simulink model "TCMSSystem"  (R2019b)
settings: configuration reference "ConfigSet_TCMSSystem_Reference" (kept outside this file)
model workspace (MAT data in the model file):
  Prm_TCMSSystem : Simulink.Parameter (value not decoded)
  SampleTime = 0.05
symbols that are objects in the model workspace (value not decoded): Prm_TCMSSystem
undefined symbols (not defined in the file): ADDIntervention, AK1Status, AK2Status, AKContactorStatus, AllDoorsClosed, AllLeftDoorsClosed, AllRightDoorsClosed, APS1Fault, APS1Isolated, APS1OutputVoltage, APS1Status, APS2Fault, APS2Isolated, APS2OutputVoltage, APS2Status, APSKAKContactor, ASCOEnd1, ASCOEnd2, ATBMode, ATCBypassMode, ATCStatusNotOK, ATOMode, ATPLowSpeedCutoutStatus, ATPMode, AuxCompressor, BatteryCurrent, BatteryIsolationContactor, BatteryTemperature, BatteryVoltage, BCG1Fault, BCG1Isolated, BCG1IsolationFailed, BCG1OutputCurrent, BCG1Status, BCG2Fault, BCG2Isolated, BCG2OutputCurrent, BCG2Status, BCGOutputVoltage, BECU1AxleLockedWheelSet1, BECU2AxleLockedWheelSet2, BECUFaulty, BECUMajorFault, BECUMinorFault, BECUStatus, BIC1Inside, BIC1Outside, BIC2Inside, BIC2Outside, Bogie, Bogie1WSPStatus, Bogie2WSPStatus, BogieFaulty, BogieIsolationStatus, BogieSupportedMass, BrakeCylinderPressureGauge, BrakeLoopCBTripped, BrakeLoopOpenTL, BrakeTrainLineStatus, BrakingDemand ... (+215)
libraries: TimersLib x257, simulink x137, LatchesLib x42, VectorOperationsLib x15, TestBenchLib x12, MathOperationsLib x2, FiltersLib x1
(part 13 of 16)

== system TCMSSystem/TCMSSystemPerVehicle/EnabledTCMSVehicle/OutputsPacking/TCMSDisplayOutputs/TCMSMessageEvents/DoorSystemFaults/Associated TCMS Fault ID121 ==
  State : Inport
  Bus Creator1 : BusCreator  Inputs=2  OutDataTypeStr=Bus: BD_TCMSSystem_Out_Vehicle_Display_Message  NonVirtualBus=on
  Constant : Constant  Value=MessageID
  Data Type Conversion : DataTypeConversion
  Message : Outport  VectorParamsAs1DForOutWhenUnconnected=off
  wires:
  Data Type Conversion/1 -> Bus Creator1/2  "MessageStatus"
  Constant/1 -> Bus Creator1/1  "MessageID"
  State/1 -> Data Type Conversion/1
  Bus Creator1/1 -> Message/1

== system TCMSSystem/TCMSSystemPerVehicle/EnabledTCMSVehicle/OutputsPacking/TCMSDisplayOutputs/TCMSMessageEvents/DoorSystemFaults/Associated TCMS Fault ID122 ==
  State : Inport
  Bus Creator1 : BusCreator  Inputs=2  OutDataTypeStr=Bus: BD_TCMSSystem_Out_Vehicle_Display_Message  NonVirtualBus=on
  Constant : Constant  Value=MessageID
  Data Type Conversion : DataTypeConversion
  Message : Outport  VectorParamsAs1DForOutWhenUnconnected=off
  wires:
  Bus Creator1/1 -> Message/1
  State/1 -> Data Type Conversion/1
  Constant/1 -> Bus Creator1/1  "MessageID"
  Data Type Conversion/1 -> Bus Creator1/2  "MessageStatus"

== system TCMSSystem/TCMSSystemPerVehicle/EnabledTCMSVehicle/OutputsPacking/TCMSDisplayOutputs/TCMSMessageEvents/DoorSystemFaults/Associated TCMS Fault ID123 ==
  State : Inport
  Bus Creator1 : BusCreator  Inputs=2  OutDataTypeStr=Bus: BD_TCMSSystem_Out_Vehicle_Display_Message  NonVirtualBus=on
  Constant : Constant  Value=MessageID
  Data Type Conversion : DataTypeConversion
  Message : Outport  VectorParamsAs1DForOutWhenUnconnected=off
  wires:
  Data Type Conversion/1 -> Bus Creator1/2  "MessageStatus"
  Constant/1 -> Bus Creator1/1  "MessageID"
  State/1 -> Data Type Conversion/1
  Bus Creator1/1 -> Message/1

== system TCMSSystem/TCMSSystemPerVehicle/EnabledTCMSVehicle/OutputsPacking/TCMSDisplayOutputs/TCMSMessageEvents/DoorSystemFaults/Associated TCMS Fault ID124 ==
  State : Inport
  Bus Creator1 : BusCreator  Inputs=2  OutDataTypeStr=Bus: BD_TCMSSystem_Out_Vehicle_Display_Message  NonVirtualBus=on
  Constant : Constant  Value=MessageID
  Data Type Conversion : DataTypeConversion
  Message : Outport  VectorParamsAs1DForOutWhenUnconnected=off
  wires:
  Data Type Conversion/1 -> Bus Creator1/2  "MessageStatus"
  Constant/1 -> Bus Creator1/1  "MessageID"
  State/1 -> Data Type Conversion/1
  Bus Creator1/1 -> Message/1

== system TCMSSystem/TCMSSystemPerVehicle/EnabledTCMSVehicle/OutputsPacking/TCMSDisplayOutputs/TCMSMessageEvents/DoorSystemFaults/Associated TCMS Fault ID125 ==
  State : Inport
  Bus Creator1 : BusCreator  Inputs=2  OutDataTypeStr=Bus: BD_TCMSSystem_Out_Vehicle_Display_Message  NonVirtualBus=on
  Constant : Constant  Value=MessageID
  Data Type Conversion : DataTypeConversion
  Message : Outport  VectorParamsAs1DForOutWhenUnconnected=off
  wires:
  Data Type Conversion/1 -> Bus Creator1/2  "MessageStatus"
  Constant/1 -> Bus Creator1/1  "MessageID"
  State/1 -> Data Type Conversion/1
  Bus Creator1/1 -> Message/1

== system TCMSSystem/TCMSSystemPerVehicle/EnabledTCMSVehicle/OutputsPacking/TCMSDisplayOutputs/TCMSMessageEvents/DoorSystemFaults/Associated TCMS Fault ID126 ==
  State : Inport
  Bus Creator1 : BusCreator  Inputs=2  OutDataTypeStr=Bus: BD_TCMSSystem_Out_Vehicle_Display_Message  NonVirtualBus=on
  Constant : Constant  Value=MessageID
  Data Type Conversion : DataTypeConversion
  Message : Outport  VectorParamsAs1DForOutWhenUnconnected=off
  wires:
  Data Type Conversion/1 -> Bus Creator1/2  "MessageStatus"
  Constant/1 -> Bus Creator1/1  "MessageID"
  State/1 -> Data Type Conversion/1
  Bus Creator1/1 -> Message/1

== system TCMSSystem/TCMSSystemPerVehicle/EnabledTCMSVehicle/OutputsPacking/TCMSDisplayOutputs/TCMSMessageEvents/DoorSystemFaults/Associated TCMS Fault ID127 ==
  State : Inport
  Bus Creator1 : BusCreator  Inputs=2  OutDataTypeStr=Bus: BD_TCMSSystem_Out_Vehicle_Display_Message  NonVirtualBus=on
  Constant : Constant  Value=MessageID
  Data Type Conversion : DataTypeConversion
  Message : Outport  VectorParamsAs1DForOutWhenUnconnected=off
  wires:
  Data Type Conversion/1 -> Bus Creator1/2  "MessageStatus"
  Constant/1 -> Bus Creator1/1  "MessageID"
  State/1 -> Data Type Conversion/1
  Bus Creator1/1 -> Message/1

== system TCMSSystem/TCMSSystemPerVehicle/EnabledTCMSVehicle/OutputsPacking/TCMSDisplayOutputs/TCMSMessageEvents/DoorSystemFaults/Associated TCMS Fault ID128 ==
  State : Inport
  Bus Creator1 : BusCreator  Inputs=2  OutDataTypeStr=Bus: BD_TCMSSystem_Out_Vehicle_Display_Message  NonVirtualBus=on
  Constant : Constant  Value=MessageID
  Data Type Conversion : DataTypeConversion
  Message : Outport  VectorParamsAs1DForOutWhenUnconnected=off
  wires:
  Bus Creator1/1 -> Message/1
  State/1 -> Data Type Conversion/1
  Constant/1 -> Bus Creator1/1  "MessageID"
  Data Type Conversion/1 -> Bus Creator1/2  "MessageStatus"

== system TCMSSystem/TCMSSystemPerVehicle/EnabledTCMSVehicle/OutputsPacking/TCMSDisplayOutputs/TCMSMessageEvents/DoorSystemFaults/Associated TCMS Fault ID129 ==
  State : Inport
  Bus Creator1 : BusCreator  Inputs=2  OutDataTypeStr=Bus: BD_TCMSSystem_Out_Vehicle_Display_Message  NonVirtualBus=on
  Constant : Constant  Value=MessageID
  Data Type Conversion : DataTypeConversion
  Message : Outport  VectorParamsAs1DForOutWhenUnconnected=off
  wires:
  Bus Creator1/1 -> Message/1
  State/1 -> Data Type Conversion/1
  Constant/1 -> Bus Creator1/1  "MessageID"
  Data Type Conversion/1 -> Bus Creator1/2  "MessageStatus"

== system TCMSSystem/TCMSSystemPerVehicle/EnabledTCMSVehicle/OutputsPacking/TCMSDisplayOutputs/TCMSMessageEvents/DoorSystemFaults/Associated TCMS Fault ID13 ==
  State : Inport
  Bus Creator1 : BusCreator  Inputs=2  OutDataTypeStr=Bus: BD_TCMSSystem_Out_Vehicle_Display_Message  NonVirtualBus=on
  Constant : Constant  Value=MessageID
  Data Type Conversion : DataTypeConversion
  Message : Outport  VectorParamsAs1DForOutWhenUnconnected=off
  wires:
  Bus Creator1/1 -> Message/1
  State/1 -> Data Type Conversion/1
  Constant/1 -> Bus Creator1/1  "MessageID"
  Data Type Conversion/1 -> Bus Creator1/2  "MessageStatus"

== system TCMSSystem/TCMSSystemPerVehicle/EnabledTCMSVehicle/OutputsPacking/TCMSDisplayOutputs/TCMSMessageEvents/DoorSystemFaults/Associated TCMS Fault ID130 ==
  State : Inport
  Bus Creator1 : BusCreator  Inputs=2  OutDataTypeStr=Bus: BD_TCMSSystem_Out_Vehicle_Display_Message  NonVirtualBus=on
  Constant : Constant  Value=MessageID
  Data Type Conversion : DataTypeConversion
  Message : Outport  VectorParamsAs1DForOutWhenUnconnected=off
  wires:
  Data Type Conversion/1 -> Bus Creator1/2  "MessageStatus"
  Constant/1 -> Bus Creator1/1  "MessageID"
  State/1 -> Data Type Conversion/1
  Bus Creator1/1 -> Message/1

== system TCMSSystem/TCMSSystemPerVehicle/EnabledTCMSVehicle/OutputsPacking/TCMSDisplayOutputs/TCMSMessageEvents/DoorSystemFaults/Associated TCMS Fault ID131 ==
  State : Inport
  Bus Creator1 : BusCreator  Inputs=2  OutDataTypeStr=Bus: BD_TCMSSystem_Out_Vehicle_Display_Message  NonVirtualBus=on
  Constant : Constant  Value=MessageID
  Data Type Conversion : DataTypeConversion
  Message : Outport  VectorParamsAs1DForOutWhenUnconnected=off
  wires:
  Data Type Conversion/1 -> Bus Creator1/2  "MessageStatus"
  Constant/1 -> Bus Creator1/1  "MessageID"
  State/1 -> Data Type Conversion/1
  Bus Creator1/1 -> Message/1

== system TCMSSystem/TCMSSystemPerVehicle/EnabledTCMSVehicle/OutputsPacking/TCMSDisplayOutputs/TCMSMessageEvents/DoorSystemFaults/Associated TCMS Fault ID132 ==
  State : Inport
  Bus Creator1 : BusCreator  Inputs=2  OutDataTypeStr=Bus: BD_TCMSSystem_Out_Vehicle_Display_Message  NonVirtualBus=on
  Constant : Constant  Value=MessageID
  Data Type Conversion : DataTypeConversion
  Message : Outport  VectorParamsAs1DForOutWhenUnconnected=off
  wires:
  Data Type Conversion/1 -> Bus Creator1/2  "MessageStatus"
  Constant/1 -> Bus Creator1/1  "MessageID"
  State/1 -> Data Type Conversion/1
  Bus Creator1/1 -> Message/1

== system TCMSSystem/TCMSSystemPerVehicle/EnabledTCMSVehicle/OutputsPacking/TCMSDisplayOutputs/TCMSMessageEvents/DoorSystemFaults/Associated TCMS Fault ID133 ==
  State : Inport
  Bus Creator1 : BusCreator  Inputs=2  OutDataTypeStr=Bus: BD_TCMSSystem_Out_Vehicle_Display_Message  NonVirtualBus=on
  Constant : Constant  Value=MessageID
  Data Type Conversion : DataTypeConversion
  Message : Outport  VectorParamsAs1DForOutWhenUnconnected=off
  wires:
  Data Type Conversion/1 -> Bus Creator1/2  "MessageStatus"
  Constant/1 -> Bus Creator1/1  "MessageID"
  State/1 -> Data Type Conversion/1
  Bus Creator1/1 -> Message/1

== system TCMSSystem/TCMSSystemPerVehicle/EnabledTCMSVehicle/OutputsPacking/TCMSDisplayOutputs/TCMSMessageEvents/DoorSystemFaults/Associated TCMS Fault ID134 ==
  State : Inport
  Bus Creator1 : BusCreator  Inputs=2  OutDataTypeStr=Bus: BD_TCMSSystem_Out_Vehicle_Display_Message  NonVirtualBus=on
  Constant : Constant  Value=MessageID
  Data Type Conversion : DataTypeConversion
  Message : Outport  VectorParamsAs1DForOutWhenUnconnected=off
  wires:
  Data Type Conversion/1 -> Bus Creator1/2  "MessageStatus"
  Constant/1 -> Bus Creator1/1  "MessageID"
  State/1 -> Data Type Conversion/1
  Bus Creator1/1 -> Message/1

== system TCMSSystem/TCMSSystemPerVehicle/EnabledTCMSVehicle/OutputsPacking/TCMSDisplayOutputs/TCMSMessageEvents/DoorSystemFaults/Associated TCMS Fault ID135 ==
  State : Inport
  Bus Creator1 : BusCreator  Inputs=2  OutDataTypeStr=Bus: BD_TCMSSystem_Out_Vehicle_Display_Message  NonVirtualBus=on
  Constant : Constant  Value=MessageID
  Data Type Conversion : DataTypeConversion
  Message : Outport  VectorParamsAs1DForOutWhenUnconnected=off
  wires:
  Bus Creator1/1 -> Message/1
  State/1 -> Data Type Conversion/1
  Constant/1 -> Bus Creator1/1  "MessageID"
  Data Type Conversion/1 -> Bus Creator1/2  "MessageStatus"

== system TCMSSystem/TCMSSystemPerVehicle/EnabledTCMSVehicle/OutputsPacking/TCMSDisplayOutputs/TCMSMessageEvents/DoorSystemFaults/Associated TCMS Fault ID14 ==
  State : Inport
  Bus Creator1 : BusCreator  Inputs=2  OutDataTypeStr=Bus: BD_TCMSSystem_Out_Vehicle_Display_Message  NonVirtualBus=on
  Constant : Constant  Value=MessageID
  Data Type Conversion : DataTypeConversion
  Message : Outport  VectorParamsAs1DForOutWhenUnconnected=off
  wires:
  Bus Creator1/1 -> Message/1
  State/1 -> Data Type Conversion/1
  Constant/1 -> Bus Creator1/1  "MessageID"
  Data Type Conversion/1 -> Bus Creator1/2  "MessageStatus"

== system TCMSSystem/TCMSSystemPerVehicle/EnabledTCMSVehicle/OutputsPacking/TCMSDisplayOutputs/TCMSMessageEvents/DoorSystemFaults/Associated TCMS Fault ID15 ==
  State : Inport
  Bus Creator1 : BusCreator  Inputs=2  OutDataTypeStr=Bus: BD_TCMSSystem_Out_Vehicle_Display_Message  NonVirtualBus=on
  Constant : Constant  Value=MessageID
  Data Type Conversion : DataTypeConversion
  Message : Outport  VectorParamsAs1DForOutWhenUnconnected=off
  wires:
  Bus Creator1/1 -> Message/1
  State/1 -> Data Type Conversion/1
  Constant/1 -> Bus Creator1/1  "MessageID"
  Data Type Conversion/1 -> Bus Creator1/2  "MessageStatus"

== system TCMSSystem/TCMSSystemPerVehicle/EnabledTCMSVehicle/OutputsPacking/TCMSDisplayOutputs/TCMSMessageEvents/DoorSystemFaults/Associated TCMS Fault ID16 ==
  State : Inport
  Bus Creator1 : BusCreator  Inputs=2  OutDataTypeStr=Bus: BD_TCMSSystem_Out_Vehicle_Display_Message  NonVirtualBus=on
  Constant : Constant  Value=MessageID
  Data Type Conversion : DataTypeConversion
  Message : Outport  VectorParamsAs1DForOutWhenUnconnected=off
  wires:
  Bus Creator1/1 -> Message/1
  State/1 -> Data Type Conversion/1
  Constant/1 -> Bus Creator1/1  "MessageID"
  Data Type Conversion/1 -> Bus Creator1/2  "MessageStatus"

== system TCMSSystem/TCMSSystemPerVehicle/EnabledTCMSVehicle/OutputsPacking/TCMSDisplayOutputs/TCMSMessageEvents/DoorSystemFaults/Associated TCMS Fault ID17 ==
  State : Inport
  Bus Creator1 : BusCreator  Inputs=2  OutDataTypeStr=Bus: BD_TCMSSystem_Out_Vehicle_Display_Message  NonVirtualBus=on
  Constant : Constant  Value=MessageID
  Data Type Conversion : DataTypeConversion
  Message : Outport  VectorParamsAs1DForOutWhenUnconnected=off
  wires:
  Bus Creator1/1 -> Message/1
  State/1 -> Data Type Conversion/1
  Constant/1 -> Bus Creator1/1  "MessageID"
  Data Type Conversion/1 -> Bus Creator1/2  "MessageStatus"

== system TCMSSystem/TCMSSystemPerVehicle/EnabledTCMSVehicle/OutputsPacking/TCMSDisplayOutputs/TCMSMessageEvents/DoorSystemFaults/Associated TCMS Fault ID18 ==
  State : Inport
  Bus Creator1 : BusCreator  Inputs=2  OutDataTypeStr=Bus: BD_TCMSSystem_Out_Vehicle_Display_Message  NonVirtualBus=on
  Constant : Constant  Value=MessageID
  Data Type Conversion : DataTypeConversion
  Message : Outport  VectorParamsAs1DForOutWhenUnconnected=off
  wires:
  Bus Creator1/1 -> Message/1
  State/1 -> Data Type Conversion/1
  Constant/1 -> Bus Creator1/1  "MessageID"
  Data Type Conversion/1 -> Bus Creator1/2  "MessageStatus"

== system TCMSSystem/TCMSSystemPerVehicle/EnabledTCMSVehicle/OutputsPacking/TCMSDisplayOutputs/TCMSMessageEvents/DoorSystemFaults/Associated TCMS Fault ID19 ==
  State : Inport
  Bus Creator1 : BusCreator  Inputs=2  OutDataTypeStr=Bus: BD_TCMSSystem_Out_Vehicle_Display_Message  NonVirtualBus=on
  Constant : Constant  Value=MessageID
  Data Type Conversion : DataTypeConversion
  Message : Outport  VectorParamsAs1DForOutWhenUnconnected=off
  wires:
  Bus Creator1/1 -> Message/1
  State/1 -> Data Type Conversion/1
  Constant/1 -> Bus Creator1/1  "MessageID"
  Data Type Conversion/1 -> Bus Creator1/2  "MessageStatus"

== system TCMSSystem/TCMSSystemPerVehicle/EnabledTCMSVehicle/OutputsPacking/TCMSDisplayOutputs/TCMSMessageEvents/DoorSystemFaults/Associated TCMS Fault ID2 ==
  State : Inport
  Bus Creator1 : BusCreator  Inputs=2  OutDataTypeStr=Bus: BD_TCMSSystem_Out_Vehicle_Display_Message  NonVirtualBus=on
  Constant : Constant  Value=MessageID
  Data Type Conversion : DataTypeConversion
  Message : Outport  VectorParamsAs1DForOutWhenUnconnected=off
  wires:
  Data Type Conversion/1 -> Bus Creator1/2  "MessageStatus"
  Constant/1 -> Bus Creator1/1  "MessageID"
  State/1 -> Data Type Conversion/1
  Bus Creator1/1 -> Message/1

== system TCMSSystem/TCMSSystemPerVehicle/EnabledTCMSVehicle/OutputsPacking/TCMSDisplayOutputs/TCMSMessageEvents/DoorSystemFaults/Associated TCMS Fault ID20 ==
  State : Inport
  Bus Creator1 : BusCreator  Inputs=2  OutDataTypeStr=Bus: BD_TCMSSystem_Out_Vehicle_Display_Message  NonVirtualBus=on
  Constant : Constant  Value=MessageID
  Data Type Conversion : DataTypeConversion
  Message : Outport  VectorParamsAs1DForOutWhenUnconnected=off
  wires:
  Data Type Conversion/1 -> Bus Creator1/2  "MessageStatus"
  Constant/1 -> Bus Creator1/1  "MessageID"
  State/1 -> Data Type Conversion/1
  Bus Creator1/1 -> Message/1

== system TCMSSystem/TCMSSystemPerVehicle/EnabledTCMSVehicle/OutputsPacking/TCMSDisplayOutputs/TCMSMessageEvents/DoorSystemFaults/Associated TCMS Fault ID21 ==
  State : Inport
  Bus Creator1 : BusCreator  Inputs=2  OutDataTypeStr=Bus: BD_TCMSSystem_Out_Vehicle_Display_Message  NonVirtualBus=on
  Constant : Constant  Value=MessageID
  Data Type Conversion : DataTypeConversion
  Message : Outport  VectorParamsAs1DForOutWhenUnconnected=off
  wires:
  Data Type Conversion/1 -> Bus Creator1/2  "MessageStatus"
  Constant/1 -> Bus Creator1/1  "MessageID"
  State/1 -> Data Type Conversion/1
  Bus Creator1/1 -> Message/1

== system TCMSSystem/TCMSSystemPerVehicle/EnabledTCMSVehicle/OutputsPacking/TCMSDisplayOutputs/TCMSMessageEvents/DoorSystemFaults/Associated TCMS Fault ID22 ==
  State : Inport
  Bus Creator1 : BusCreator  Inputs=2  OutDataTypeStr=Bus: BD_TCMSSystem_Out_Vehicle_Display_Message  NonVirtualBus=on
  Constant : Constant  Value=MessageID
  Data Type Conversion : DataTypeConversion
  Message : Outport  VectorParamsAs1DForOutWhenUnconnected=off
  wires:
  Data Type Conversion/1 -> Bus Creator1/2  "MessageStatus"
  Constant/1 -> Bus Creator1/1  "MessageID"
  State/1 -> Data Type Conversion/1
  Bus Creator1/1 -> Message/1

== system TCMSSystem/TCMSSystemPerVehicle/EnabledTCMSVehicle/OutputsPacking/TCMSDisplayOutputs/TCMSMessageEvents/DoorSystemFaults/Associated TCMS Fault ID23 ==
  State : Inport
  Bus Creator1 : BusCreator  Inputs=2  OutDataTypeStr=Bus: BD_TCMSSystem_Out_Vehicle_Display_Message  NonVirtualBus=on
  Constant : Constant  Value=MessageID
  Data Type Conversion : DataTypeConversion
  Message : Outport  VectorParamsAs1DForOutWhenUnconnected=off
  wires:
  Data Type Conversion/1 -> Bus Creator1/2  "MessageStatus"
  Constant/1 -> Bus Creator1/1  "MessageID"
  State/1 -> Data Type Conversion/1
  Bus Creator1/1 -> Message/1

== system TCMSSystem/TCMSSystemPerVehicle/EnabledTCMSVehicle/OutputsPacking/TCMSDisplayOutputs/TCMSMessageEvents/DoorSystemFaults/Associated TCMS Fault ID24 ==
  State : Inport
  Bus Creator1 : BusCreator  Inputs=2  OutDataTypeStr=Bus: BD_TCMSSystem_Out_Vehicle_Display_Message  NonVirtualBus=on
  Constant : Constant  Value=MessageID
  Data Type Conversion : DataTypeConversion
  Message : Outport  VectorParamsAs1DForOutWhenUnconnected=off
  wires:
  Data Type Conversion/1 -> Bus Creator1/2  "MessageStatus"
  Constant/1 -> Bus Creator1/1  "MessageID"
  State/1 -> Data Type Conversion/1
  Bus Creator1/1 -> Message/1

== system TCMSSystem/TCMSSystemPerVehicle/EnabledTCMSVehicle/OutputsPacking/TCMSDisplayOutputs/TCMSMessageEvents/DoorSystemFaults/Associated TCMS Fault ID25 ==
  State : Inport
  Bus Creator1 : BusCreator  Inputs=2  OutDataTypeStr=Bus: BD_TCMSSystem_Out_Vehicle_Display_Message  NonVirtualBus=on
  Constant : Constant  Value=MessageID
  Data Type Conversion : DataTypeConversion
  Message : Outport  VectorParamsAs1DForOutWhenUnconnected=off
  wires:
  Data Type Conversion/1 -> Bus Creator1/2  "MessageStatus"
  Constant/1 -> Bus Creator1/1  "MessageID"
  State/1 -> Data Type Conversion/1
  Bus Creator1/1 -> Message/1

== system TCMSSystem/TCMSSystemPerVehicle/EnabledTCMSVehicle/OutputsPacking/TCMSDisplayOutputs/TCMSMessageEvents/DoorSystemFaults/Associated TCMS Fault ID26 ==
  State : Inport
  Bus Creator1 : BusCreator  Inputs=2  OutDataTypeStr=Bus: BD_TCMSSystem_Out_Vehicle_Display_Message  NonVirtualBus=on
  Constant : Constant  Value=MessageID
  Data Type Conversion : DataTypeConversion
  Message : Outport  VectorParamsAs1DForOutWhenUnconnected=off
  wires:
  Data Type Conversion/1 -> Bus Creator1/2  "MessageStatus"
  Constant/1 -> Bus Creator1/1  "MessageID"
  State/1 -> Data Type Conversion/1
  Bus Creator1/1 -> Message/1

== system TCMSSystem/TCMSSystemPerVehicle/EnabledTCMSVehicle/OutputsPacking/TCMSDisplayOutputs/TCMSMessageEvents/DoorSystemFaults/Associated TCMS Fault ID27 ==
  State : Inport
  Bus Creator1 : BusCreator  Inputs=2  OutDataTypeStr=Bus: BD_TCMSSystem_Out_Vehicle_Display_Message  NonVirtualBus=on
  Constant : Constant  Value=MessageID
  Data Type Conversion : DataTypeConversion
  Message : Outport  VectorParamsAs1DForOutWhenUnconnected=off
  wires:
  Data Type Conversion/1 -> Bus Creator1/2  "MessageStatus"
  Constant/1 -> Bus Creator1/1  "MessageID"
  State/1 -> Data Type Conversion/1
  Bus Creator1/1 -> Message/1

== system TCMSSystem/TCMSSystemPerVehicle/EnabledTCMSVehicle/OutputsPacking/TCMSDisplayOutputs/TCMSMessageEvents/DoorSystemFaults/Associated TCMS Fault ID28 ==
  State : Inport
  Bus Creator1 : BusCreator  Inputs=2  OutDataTypeStr=Bus: BD_TCMSSystem_Out_Vehicle_Display_Message  NonVirtualBus=on
  Constant : Constant  Value=MessageID
  Data Type Conversion : DataTypeConversion
  Message : Outport  VectorParamsAs1DForOutWhenUnconnected=off
  wires:
  Data Type Conversion/1 -> Bus Creator1/2  "MessageStatus"
  Constant/1 -> Bus Creator1/1  "MessageID"
  State/1 -> Data Type Conversion/1
  Bus Creator1/1 -> Message/1

== system TCMSSystem/TCMSSystemPerVehicle/EnabledTCMSVehicle/OutputsPacking/TCMSDisplayOutputs/TCMSMessageEvents/DoorSystemFaults/Associated TCMS Fault ID29 ==
  State : Inport
  Bus Creator1 : BusCreator  Inputs=2  OutDataTypeStr=Bus: BD_TCMSSystem_Out_Vehicle_Display_Message  NonVirtualBus=on
  Constant : Constant  Value=MessageID
  Data Type Conversion : DataTypeConversion
  Message : Outport  VectorParamsAs1DForOutWhenUnconnected=off
  wires:
  Data Type Conversion/1 -> Bus Creator1/2  "MessageStatus"
  Constant/1 -> Bus Creator1/1  "MessageID"
  State/1 -> Data Type Conversion/1
  Bus Creator1/1 -> Message/1

== system TCMSSystem/TCMSSystemPerVehicle/EnabledTCMSVehicle/OutputsPacking/TCMSDisplayOutputs/TCMSMessageEvents/DoorSystemFaults/Associated TCMS Fault ID3 ==
  State : Inport
  Bus Creator1 : BusCreator  Inputs=2  OutDataTypeStr=Bus: BD_TCMSSystem_Out_Vehicle_Display_Message  NonVirtualBus=on
  Constant : Constant  Value=MessageID
  Data Type Conversion : DataTypeConversion
  Message : Outport  VectorParamsAs1DForOutWhenUnconnected=off
  wires:
  Data Type Conversion/1 -> Bus Creator1/2  "MessageStatus"
  Constant/1 -> Bus Creator1/1  "MessageID"
  State/1 -> Data Type Conversion/1
  Bus Creator1/1 -> Message/1

== system TCMSSystem/TCMSSystemPerVehicle/EnabledTCMSVehicle/OutputsPacking/TCMSDisplayOutputs/TCMSMessageEvents/DoorSystemFaults/Associated TCMS Fault ID30 ==
  State : Inport
  Bus Creator1 : BusCreator  Inputs=2  OutDataTypeStr=Bus: BD_TCMSSystem_Out_Vehicle_Display_Message  NonVirtualBus=on
  Constant : Constant  Value=MessageID
  Data Type Conversion : DataTypeConversion
  Message : Outport  VectorParamsAs1DForOutWhenUnconnected=off
  wires:
  Bus Creator1/1 -> Message/1
  State/1 -> Data Type Conversion/1
  Constant/1 -> Bus Creator1/1  "MessageID"
  Data Type Conversion/1 -> Bus Creator1/2  "MessageStatus"

== system TCMSSystem/TCMSSystemPerVehicle/EnabledTCMSVehicle/OutputsPacking/TCMSDisplayOutputs/TCMSMessageEvents/DoorSystemFaults/Associated TCMS Fault ID31 ==
  State : Inport
  Bus Creator1 : BusCreator  Inputs=2  OutDataTypeStr=Bus: BD_TCMSSystem_Out_Vehicle_Display_Message  NonVirtualBus=on
  Constant : Constant  Value=MessageID
  Data Type Conversion : DataTypeConversion
  Message : Outport  VectorParamsAs1DForOutWhenUnconnected=off
  wires:
  Bus Creator1/1 -> Message/1
  State/1 -> Data Type Conversion/1
  Constant/1 -> Bus Creator1/1  "MessageID"
  Data Type Conversion/1 -> Bus Creator1/2  "MessageStatus"

== system TCMSSystem/TCMSSystemPerVehicle/EnabledTCMSVehicle/OutputsPacking/TCMSDisplayOutputs/TCMSMessageEvents/DoorSystemFaults/Associated TCMS Fault ID32 ==
  State : Inport
  Bus Creator1 : BusCreator  Inputs=2  OutDataTypeStr=Bus: BD_TCMSSystem_Out_Vehicle_Display_Message  NonVirtualBus=on
  Constant : Constant  Value=MessageID
  Data Type Conversion : DataTypeConversion
  Message : Outport  VectorParamsAs1DForOutWhenUnconnected=off
  wires:
  Bus Creator1/1 -> Message/1
  State/1 -> Data Type Conversion/1
  Constant/1 -> Bus Creator1/1  "MessageID"
  Data Type Conversion/1 -> Bus Creator1/2  "MessageStatus"

== system TCMSSystem/TCMSSystemPerVehicle/EnabledTCMSVehicle/OutputsPacking/TCMSDisplayOutputs/TCMSMessageEvents/DoorSystemFaults/Associated TCMS Fault ID33 ==
  State : Inport
  Bus Creator1 : BusCreator  Inputs=2  OutDataTypeStr=Bus: BD_TCMSSystem_Out_Vehicle_Display_Message  NonVirtualBus=on
  Constant : Constant  Value=MessageID
  Data Type Conversion : DataTypeConversion
  Message : Outport  VectorParamsAs1DForOutWhenUnconnected=off
  wires:
  Bus Creator1/1 -> Message/1
  State/1 -> Data Type Conversion/1
  Constant/1 -> Bus Creator1/1  "MessageID"
  Data Type Conversion/1 -> Bus Creator1/2  "MessageStatus"

== system TCMSSystem/TCMSSystemPerVehicle/EnabledTCMSVehicle/OutputsPacking/TCMSDisplayOutputs/TCMSMessageEvents/DoorSystemFaults/Associated TCMS Fault ID34 ==
  State : Inport
  Bus Creator1 : BusCreator  Inputs=2  OutDataTypeStr=Bus: BD_TCMSSystem_Out_Vehicle_Display_Message  NonVirtualBus=on
  Constant : Constant  Value=MessageID
  Data Type Conversion : DataTypeConversion
  Message : Outport  VectorParamsAs1DForOutWhenUnconnected=off
  wires:
  Bus Creator1/1 -> Message/1
  State/1 -> Data Type Conversion/1
  Constant/1 -> Bus Creator1/1  "MessageID"
  Data Type Conversion/1 -> Bus Creator1/2  "MessageStatus"

== system TCMSSystem/TCMSSystemPerVehicle/EnabledTCMSVehicle/OutputsPacking/TCMSDisplayOutputs/TCMSMessageEvents/DoorSystemFaults/Associated TCMS Fault ID35 ==
  State : Inport
  Bus Creator1 : BusCreator  Inputs=2  OutDataTypeStr=Bus: BD_TCMSSystem_Out_Vehicle_Display_Message  NonVirtualBus=on
  Constant : Constant  Value=MessageID
  Data Type Conversion : DataTypeConversion
  Message : Outport  VectorParamsAs1DForOutWhenUnconnected=off
  wires:
  Bus Creator1/1 -> Message/1
  State/1 -> Data Type Conversion/1
  Constant/1 -> Bus Creator1/1  "MessageID"
  Data Type Conversion/1 -> Bus Creator1/2  "MessageStatus"

== system TCMSSystem/TCMSSystemPerVehicle/EnabledTCMSVehicle/OutputsPacking/TCMSDisplayOutputs/TCMSMessageEvents/DoorSystemFaults/Associated TCMS Fault ID36 ==
  State : Inport
  Bus Creator1 : BusCreator  Inputs=2  OutDataTypeStr=Bus: BD_TCMSSystem_Out_Vehicle_Display_Message  NonVirtualBus=on
  Constant : Constant  Value=MessageID
  Data Type Conversion : DataTypeConversion
  Message : Outport  VectorParamsAs1DForOutWhenUnconnected=off
  wires:
  Bus Creator1/1 -> Message/1
  State/1 -> Data Type Conversion/1
  Constant/1 -> Bus Creator1/1  "MessageID"
  Data Type Conversion/1 -> Bus Creator1/2  "MessageStatus"

== system TCMSSystem/TCMSSystemPerVehicle/EnabledTCMSVehicle/OutputsPacking/TCMSDisplayOutputs/TCMSMessageEvents/DoorSystemFaults/Associated TCMS Fault ID37 ==
  State : Inport
  Bus Creator1 : BusCreator  Inputs=2  OutDataTypeStr=Bus: BD_TCMSSystem_Out_Vehicle_Display_Message  NonVirtualBus=on
  Constant : Constant  Value=MessageID
  Data Type Conversion : DataTypeConversion
  Message : Outport  VectorParamsAs1DForOutWhenUnconnected=off
  wires:
  Bus Creator1/1 -> Message/1
  State/1 -> Data Type Conversion/1
  Constant/1 -> Bus Creator1/1  "MessageID"
  Data Type Conversion/1 -> Bus Creator1/2  "MessageStatus"

== system TCMSSystem/TCMSSystemPerVehicle/EnabledTCMSVehicle/OutputsPacking/TCMSDisplayOutputs/TCMSMessageEvents/DoorSystemFaults/Associated TCMS Fault ID38 ==
  State : Inport
  Bus Creator1 : BusCreator  Inputs=2  OutDataTypeStr=Bus: BD_TCMSSystem_Out_Vehicle_Display_Message  NonVirtualBus=on
  Constant : Constant  Value=MessageID
  Data Type Conversion : DataTypeConversion
  Message : Outport  VectorParamsAs1DForOutWhenUnconnected=off
  wires:
  Bus Creator1/1 -> Message/1
  State/1 -> Data Type Conversion/1
  Constant/1 -> Bus Creator1/1  "MessageID"
  Data Type Conversion/1 -> Bus Creator1/2  "MessageStatus"

== system TCMSSystem/TCMSSystemPerVehicle/EnabledTCMSVehicle/OutputsPacking/TCMSDisplayOutputs/TCMSMessageEvents/DoorSystemFaults/Associated TCMS Fault ID4 ==
  State : Inport
  Bus Creator1 : BusCreator  Inputs=2  OutDataTypeStr=Bus: BD_TCMSSystem_Out_Vehicle_Display_Message  NonVirtualBus=on
  Constant : Constant  Value=MessageID
  Data Type Conversion : DataTypeConversion
  Message : Outport  VectorParamsAs1DForOutWhenUnconnected=off
  wires:
  Data Type Conversion/1 -> Bus Creator1/2  "MessageStatus"
  Constant/1 -> Bus Creator1/1  "MessageID"
  State/1 -> Data Type Conversion/1
  Bus Creator1/1 -> Message/1

== system TCMSSystem/TCMSSystemPerVehicle/EnabledTCMSVehicle/OutputsPacking/TCMSDisplayOutputs/TCMSMessageEvents/DoorSystemFaults/Associated TCMS Fault ID5 ==
  State : Inport
  Bus Creator1 : BusCreator  Inputs=2  OutDataTypeStr=Bus: BD_TCMSSystem_Out_Vehicle_Display_Message  NonVirtualBus=on
  Constant : Constant  Value=MessageID
  Data Type Conversion : DataTypeConversion
  Message : Outport  VectorParamsAs1DForOutWhenUnconnected=off
  wires:
  Data Type Conversion/1 -> Bus Creator1/2  "MessageStatus"
  Constant/1 -> Bus Creator1/1  "MessageID"
  State/1 -> Data Type Conversion/1
  Bus Creator1/1 -> Message/1

== system TCMSSystem/TCMSSystemPerVehicle/EnabledTCMSVehicle/OutputsPacking/TCMSDisplayOutputs/TCMSMessageEvents/DoorSystemFaults/Associated TCMS Fault ID6 ==
  State : Inport
  Bus Creator1 : BusCreator  Inputs=2  OutDataTypeStr=Bus: BD_TCMSSystem_Out_Vehicle_Display_Message  NonVirtualBus=on
  Constant : Constant  Value=MessageID
  Data Type Conversion : DataTypeConversion
  Message : Outport  VectorParamsAs1DForOutWhenUnconnected=off
  wires:
  Data Type Conversion/1 -> Bus Creator1/2  "MessageStatus"
  Constant/1 -> Bus Creator1/1  "MessageID"
  State/1 -> Data Type Conversion/1
  Bus Creator1/1 -> Message/1

== system TCMSSystem/TCMSSystemPerVehicle/EnabledTCMSVehicle/OutputsPacking/TCMSDisplayOutputs/TCMSMessageEvents/DoorSystemFaults/Associated TCMS Fault ID7 ==
  State : Inport
  Bus Creator1 : BusCreator  Inputs=2  OutDataTypeStr=Bus: BD_TCMSSystem_Out_Vehicle_Display_Message  NonVirtualBus=on
  Constant : Constant  Value=MessageID
  Data Type Conversion : DataTypeConversion
  Message : Outport  VectorParamsAs1DForOutWhenUnconnected=off
  wires:
  Data Type Conversion/1 -> Bus Creator1/2  "MessageStatus"
  Constant/1 -> Bus Creator1/1  "MessageID"
  State/1 -> Data Type Conversion/1
  Bus Creator1/1 -> Message/1

== system TCMSSystem/TCMSSystemPerVehicle/EnabledTCMSVehicle/OutputsPacking/TCMSDisplayOutputs/TCMSMessageEvents/DoorSystemFaults/Associated TCMS Fault ID8 ==
  State : Inport
  Bus Creator1 : BusCreator  Inputs=2  OutDataTypeStr=Bus: BD_TCMSSystem_Out_Vehicle_Display_Message  NonVirtualBus=on
  Constant : Constant  Value=MessageID
  Data Type Conversion : DataTypeConversion
  Message : Outport  VectorParamsAs1DForOutWhenUnconnected=off
  wires:
  Data Type Conversion/1 -> Bus Creator1/2  "MessageStatus"
  Constant/1 -> Bus Creator1/1  "MessageID"
  State/1 -> Data Type Conversion/1
  Bus Creator1/1 -> Message/1

== system TCMSSystem/TCMSSystemPerVehicle/EnabledTCMSVehicle/OutputsPacking/TCMSDisplayOutputs/TCMSMessageEvents/DoorSystemFaults/Associated TCMS Fault ID9 ==
  State : Inport
  Bus Creator1 : BusCreator  Inputs=2  OutDataTypeStr=Bus: BD_TCMSSystem_Out_Vehicle_Display_Message  NonVirtualBus=on
  Constant : Constant  Value=MessageID
  Data Type Conversion : DataTypeConversion
  Message : Outport  VectorParamsAs1DForOutWhenUnconnected=off
  wires:
  Data Type Conversion/1 -> Bus Creator1/2  "MessageStatus"
  Constant/1 -> Bus Creator1/1  "MessageID"
  State/1 -> Data Type Conversion/1
  Bus Creator1/1 -> Message/1

== system TCMSSystem/TCMSSystemPerVehicle/EnabledTCMSVehicle/OutputsPacking/TCMSDisplayOutputs/TCMSMessageEvents/ElectricalSystemFaults/Associated TCMS Fault ID1 ==
  State : Inport
  Bus Creator1 : BusCreator  Inputs=2  OutDataTypeStr=Bus: BD_TCMSSystem_Out_Vehicle_Display_Message  NonVirtualBus=on
  Constant : Constant  Value=MessageID
  Data Type Conversion : DataTypeConversion
  Message : Outport  VectorParamsAs1DForOutWhenUnconnected=off
  wires:
  Data Type Conversion/1 -> Bus Creator1/2  "MessageStatus"
  Constant/1 -> Bus Creator1/1  "MessageID"
  State/1 -> Data Type Conversion/1
  Bus Creator1/1 -> Message/1

== system TCMSSystem/TCMSSystemPerVehicle/EnabledTCMSVehicle/OutputsPacking/TCMSDisplayOutputs/TCMSMessageEvents/ElectricalSystemFaults/Associated TCMS Fault ID10 ==
  State : Inport
  Bus Creator1 : BusCreator  Inputs=2  OutDataTypeStr=Bus: BD_TCMSSystem_Out_Vehicle_Display_Message  NonVirtualBus=on
  Constant : Constant  Value=MessageID
  Data Type Conversion : DataTypeConversion
  Message : Outport  VectorParamsAs1DForOutWhenUnconnected=off
  wires:
  Data Type Conversion/1 -> Bus Creator1/2  "MessageStatus"
  Constant/1 -> Bus Creator1/1  "MessageID"
  State/1 -> Data Type Conversion/1
  Bus Creator1/1 -> Message/1

== system TCMSSystem/TCMSSystemPerVehicle/EnabledTCMSVehicle/OutputsPacking/TCMSDisplayOutputs/TCMSMessageEvents/ElectricalSystemFaults/Associated TCMS Fault ID11 ==
  State : Inport
  Bus Creator1 : BusCreator  Inputs=2  OutDataTypeStr=Bus: BD_TCMSSystem_Out_Vehicle_Display_Message  NonVirtualBus=on
  Constant : Constant  Value=MessageID
  Data Type Conversion : DataTypeConversion
  Message : Outport  VectorParamsAs1DForOutWhenUnconnected=off
  wires:
  Bus Creator1/1 -> Message/1
  State/1 -> Data Type Conversion/1
  Constant/1 -> Bus Creator1/1  "MessageID"
  Data Type Conversion/1 -> Bus Creator1/2  "MessageStatus"

== system TCMSSystem/TCMSSystemPerVehicle/EnabledTCMSVehicle/OutputsPacking/TCMSDisplayOutputs/TCMSMessageEvents/ElectricalSystemFaults/Associated TCMS Fault ID12 ==
  State : Inport
  Bus Creator1 : BusCreator  Inputs=2  OutDataTypeStr=Bus: BD_TCMSSystem_Out_Vehicle_Display_Message  NonVirtualBus=on
  Constant : Constant  Value=MessageID
  Data Type Conversion : DataTypeConversion
  Message : Outport  VectorParamsAs1DForOutWhenUnconnected=off
  wires:
  Bus Creator1/1 -> Message/1
  State/1 -> Data Type Conversion/1
  Constant/1 -> Bus Creator1/1  "MessageID"
  Data Type Conversion/1 -> Bus Creator1/2  "MessageStatus"

== system TCMSSystem/TCMSSystemPerVehicle/EnabledTCMSVehicle/OutputsPacking/TCMSDisplayOutputs/TCMSMessageEvents/ElectricalSystemFaults/Associated TCMS Fault ID13 ==
  State : Inport
  Bus Creator1 : BusCreator  Inputs=2  OutDataTypeStr=Bus: BD_TCMSSystem_Out_Vehicle_Display_Message  NonVirtualBus=on
  Constant : Constant  Value=MessageID
  Data Type Conversion : DataTypeConversion
  Message : Outport  VectorParamsAs1DForOutWhenUnconnected=off
  wires:
  Data Type Conversion/1 -> Bus Creator1/2  "MessageStatus"
  Constant/1 -> Bus Creator1/1  "MessageID"
  State/1 -> Data Type Conversion/1
  Bus Creator1/1 -> Message/1

== system TCMSSystem/TCMSSystemPerVehicle/EnabledTCMSVehicle/OutputsPacking/TCMSDisplayOutputs/TCMSMessageEvents/ElectricalSystemFaults/Associated TCMS Fault ID14 ==
  State : Inport
  Bus Creator1 : BusCreator  Inputs=2  OutDataTypeStr=Bus: BD_TCMSSystem_Out_Vehicle_Display_Message  NonVirtualBus=on
  Constant : Constant  Value=MessageID
  Data Type Conversion : DataTypeConversion
  Message : Outport  VectorParamsAs1DForOutWhenUnconnected=off
  wires:
  Bus Creator1/1 -> Message/1
  State/1 -> Data Type Conversion/1
  Constant/1 -> Bus Creator1/1  "MessageID"
  Data Type Conversion/1 -> Bus Creator1/2  "MessageStatus"

== system TCMSSystem/TCMSSystemPerVehicle/EnabledTCMSVehicle/OutputsPacking/TCMSDisplayOutputs/TCMSMessageEvents/ElectricalSystemFaults/Associated TCMS Fault ID15 ==
  State : Inport
  Bus Creator1 : BusCreator  Inputs=2  OutDataTypeStr=Bus: BD_TCMSSystem_Out_Vehicle_Display_Message  NonVirtualBus=on
  Constant : Constant  Value=MessageID
  Data Type Conversion : DataTypeConversion
  Message : Outport  VectorParamsAs1DForOutWhenUnconnected=off
  wires:
  Data Type Conversion/1 -> Bus Creator1/2  "MessageStatus"
  Constant/1 -> Bus Creator1/1  "MessageID"
  State/1 -> Data Type Conversion/1
  Bus Creator1/1 -> Message/1

== system TCMSSystem/TCMSSystemPerVehicle/EnabledTCMSVehicle/OutputsPacking/TCMSDisplayOutputs/TCMSMessageEvents/ElectricalSystemFaults/Associated TCMS Fault ID16 ==
  State : Inport
  Bus Creator1 : BusCreator  Inputs=2  OutDataTypeStr=Bus: BD_TCMSSystem_Out_Vehicle_Display_Message  NonVirtualBus=on
  Constant : Constant  Value=MessageID
  Data Type Conversion : DataTypeConversion
  Message : Outport  VectorParamsAs1DForOutWhenUnconnected=off
  wires:
  Bus Creator1/1 -> Message/1
  State/1 -> Data Type Conversion/1
  Constant/1 -> Bus Creator1/1  "MessageID"
  Data Type Conversion/1 -> Bus Creator1/2  "MessageStatus"

== system TCMSSystem/TCMSSystemPerVehicle/EnabledTCMSVehicle/OutputsPacking/TCMSDisplayOutputs/TCMSMessageEvents/ElectricalSystemFaults/Associated TCMS Fault ID17 ==
  State : Inport
  Bus Creator1 : BusCreator  Inputs=2  OutDataTypeStr=Bus: BD_TCMSSystem_Out_Vehicle_Display_Message  NonVirtualBus=on
  Constant : Constant  Value=MessageID
  Data Type Conversion : DataTypeConversion
  Message : Outport  VectorParamsAs1DForOutWhenUnconnected=off
  wires:
  Data Type Conversion/1 -> Bus Creator1/2  "MessageStatus"
  Constant/1 -> Bus Creator1/1  "MessageID"
  State/1 -> Data Type Conversion/1
  Bus Creator1/1 -> Message/1

== system TCMSSystem/TCMSSystemPerVehicle/EnabledTCMSVehicle/OutputsPacking/TCMSDisplayOutputs/TCMSMessageEvents/ElectricalSystemFaults/Associated TCMS Fault ID18 ==
  State : Inport
  Bus Creator1 : BusCreator  Inputs=2  OutDataTypeStr=Bus: BD_TCMSSystem_Out_Vehicle_Display_Message  NonVirtualBus=on
  Constant : Constant  Value=MessageID
  Data Type Conversion : DataTypeConversion
  Message : Outport  VectorParamsAs1DForOutWhenUnconnected=off
  wires:
  Data Type Conversion/1 -> Bus Creator1/2  "MessageStatus"
  Constant/1 -> Bus Creator1/1  "MessageID"
  State/1 -> Data Type Conversion/1
  Bus Creator1/1 -> Message/1

== system TCMSSystem/TCMSSystemPerVehicle/EnabledTCMSVehicle/OutputsPacking/TCMSDisplayOutputs/TCMSMessageEvents/ElectricalSystemFaults/Associated TCMS Fault ID19 ==
  State : Inport
  Bus Creator1 : BusCreator  Inputs=2  OutDataTypeStr=Bus: BD_TCMSSystem_Out_Vehicle_Display_Message  NonVirtualBus=on
  Constant : Constant  Value=MessageID
  Data Type Conversion : DataTypeConversion
  Message : Outport  VectorParamsAs1DForOutWhenUnconnected=off
  wires:
  Bus Creator1/1 -> Message/1
  State/1 -> Data Type Conversion/1
  Constant/1 -> Bus Creator1/1  "MessageID"
  Data Type Conversion/1 -> Bus Creator1/2  "MessageStatus"

== system TCMSSystem/TCMSSystemPerVehicle/EnabledTCMSVehicle/OutputsPacking/TCMSDisplayOutputs/TCMSMessageEvents/ElectricalSystemFaults/Associated TCMS Fault ID2 ==
  State : Inport
  Bus Creator1 : BusCreator  Inputs=2  OutDataTypeStr=Bus: BD_TCMSSystem_Out_Vehicle_Display_Message  NonVirtualBus=on
  Constant : Constant  Value=MessageID
  Data Type Conversion : DataTypeConversion
  Message : Outport  VectorParamsAs1DForOutWhenUnconnected=off
  wires:
  Bus Creator1/1 -> Message/1
  State/1 -> Data Type Conversion/1
  Constant/1 -> Bus Creator1/1  "MessageID"
  Data Type Conversion/1 -> Bus Creator1/2  "MessageStatus"

== system TCMSSystem/TCMSSystemPerVehicle/EnabledTCMSVehicle/OutputsPacking/TCMSDisplayOutputs/TCMSMessageEvents/ElectricalSystemFaults/Associated TCMS Fault ID20 ==
  State : Inport
  Bus Creator1 : BusCreator  Inputs=2  OutDataTypeStr=Bus: BD_TCMSSystem_Out_Vehicle_Display_Message  NonVirtualBus=on
  Constant : Constant  Value=MessageID
  Data Type Conversion : DataTypeConversion
  Message : Outport  VectorParamsAs1DForOutWhenUnconnected=off
  wires:
  Data Type Conversion/1 -> Bus Creator1/2  "MessageStatus"
  Constant/1 -> Bus Creator1/1  "MessageID"
  State/1 -> Data Type Conversion/1
  Bus Creator1/1 -> Message/1

== system TCMSSystem/TCMSSystemPerVehicle/EnabledTCMSVehicle/OutputsPacking/TCMSDisplayOutputs/TCMSMessageEvents/ElectricalSystemFaults/Associated TCMS Fault ID21 ==
  State : Inport
  Bus Creator1 : BusCreator  Inputs=2  OutDataTypeStr=Bus: BD_TCMSSystem_Out_Vehicle_Display_Message  NonVirtualBus=on
  Constant : Constant  Value=MessageID
  Data Type Conversion : DataTypeConversion
  Message : Outport  VectorParamsAs1DForOutWhenUnconnected=off
  wires:
  Bus Creator1/1 -> Message/1
  State/1 -> Data Type Conversion/1
  Constant/1 -> Bus Creator1/1  "MessageID"
  Data Type Conversion/1 -> Bus Creator1/2  "MessageStatus"

== system TCMSSystem/TCMSSystemPerVehicle/EnabledTCMSVehicle/OutputsPacking/TCMSDisplayOutputs/TCMSMessageEvents/ElectricalSystemFaults/Associated TCMS Fault ID22 ==
  State : Inport
  Bus Creator1 : BusCreator  Inputs=2  OutDataTypeStr=Bus: BD_TCMSSystem_Out_Vehicle_Display_Message  NonVirtualBus=on
  Constant : Constant  Value=MessageID
  Data Type Conversion : DataTypeConversion
  Message : Outport  VectorParamsAs1DForOutWhenUnconnected=off
  wires:
  Bus Creator1/1 -> Message/1
  State/1 -> Data Type Conversion/1
  Constant/1 -> Bus Creator1/1  "MessageID"
  Data Type Conversion/1 -> Bus Creator1/2  "MessageStatus"

== system TCMSSystem/TCMSSystemPerVehicle/EnabledTCMSVehicle/OutputsPacking/TCMSDisplayOutputs/TCMSMessageEvents/ElectricalSystemFaults/Associated TCMS Fault ID23 ==
  State : Inport
  Bus Creator1 : BusCreator  Inputs=2  OutDataTypeStr=Bus: BD_TCMSSystem_Out_Vehicle_Display_Message  NonVirtualBus=on
  Constant : Constant  Value=MessageID
  Data Type Conversion : DataTypeConversion
  Message : Outport  VectorParamsAs1DForOutWhenUnconnected=off
  wires:
  Bus Creator1/1 -> Message/1
  State/1 -> Data Type Conversion/1
  Constant/1 -> Bus Creator1/1  "MessageID"
  Data Type Conversion/1 -> Bus Creator1/2  "MessageStatus"

== system TCMSSystem/TCMSSystemPerVehicle/EnabledTCMSVehicle/OutputsPacking/TCMSDisplayOutputs/TCMSMessageEvents/ElectricalSystemFaults/Associated TCMS Fault ID24 ==
  State : Inport
  Bus Creator1 : BusCreator  Inputs=2  OutDataTypeStr=Bus: BD_TCMSSystem_Out_Vehicle_Display_Message  NonVirtualBus=on
  Constant : Constant  Value=MessageID
  Data Type Conversion : DataTypeConversion
  Message : Outport  VectorParamsAs1DForOutWhenUnconnected=off
  wires:
  Data Type Conversion/1 -> Bus Creator1/2  "MessageStatus"
  Constant/1 -> Bus Creator1/1  "MessageID"
  State/1 -> Data Type Conversion/1
  Bus Creator1/1 -> Message/1

== system TCMSSystem/TCMSSystemPerVehicle/EnabledTCMSVehicle/OutputsPacking/TCMSDisplayOutputs/TCMSMessageEvents/ElectricalSystemFaults/Associated TCMS Fault ID25 ==
  State : Inport
  Bus Creator1 : BusCreator  Inputs=2  OutDataTypeStr=Bus: BD_TCMSSystem_Out_Vehicle_Display_Message  NonVirtualBus=on
  Constant : Constant  Value=MessageID
  Data Type Conversion : DataTypeConversion
  Message : Outport  VectorParamsAs1DForOutWhenUnconnected=off
  wires:
  Data Type Conversion/1 -> Bus Creator1/2  "MessageStatus"
  Constant/1 -> Bus Creator1/1  "MessageID"
  State/1 -> Data Type Conversion/1
  Bus Creator1/1 -> Message/1

== system TCMSSystem/TCMSSystemPerVehicle/EnabledTCMSVehicle/OutputsPacking/TCMSDisplayOutputs/TCMSMessageEvents/ElectricalSystemFaults/Associated TCMS Fault ID26 ==
  State : Inport
  Bus Creator1 : BusCreator  Inputs=2  OutDataTypeStr=Bus: BD_TCMSSystem_Out_Vehicle_Display_Message  NonVirtualBus=on
  Constant : Constant  Value=MessageID
  Data Type Conversion : DataTypeConversion
  Message : Outport  VectorParamsAs1DForOutWhenUnconnected=off
  wires:
  Bus Creator1/1 -> Message/1
  State/1 -> Data Type Conversion/1
  Constant/1 -> Bus Creator1/1  "MessageID"
  Data Type Conversion/1 -> Bus Creator1/2  "MessageStatus"

== system TCMSSystem/TCMSSystemPerVehicle/EnabledTCMSVehicle/OutputsPacking/TCMSDisplayOutputs/TCMSMessageEvents/ElectricalSystemFaults/Associated TCMS Fault ID27 ==
  State : Inport
  Bus Creator1 : BusCreator  Inputs=2  OutDataTypeStr=Bus: BD_TCMSSystem_Out_Vehicle_Display_Message  NonVirtualBus=on
  Constant : Constant  Value=MessageID
  Data Type Conversion : DataTypeConversion
  Message : Outport  VectorParamsAs1DForOutWhenUnconnected=off
  wires:
  Data Type Conversion/1 -> Bus Creator1/2  "MessageStatus"
  Constant/1 -> Bus Creator1/1  "MessageID"
  State/1 -> Data Type Conversion/1
  Bus Creator1/1 -> Message/1

== system TCMSSystem/TCMSSystemPerVehicle/EnabledTCMSVehicle/OutputsPacking/TCMSDisplayOutputs/TCMSMessageEvents/ElectricalSystemFaults/Associated TCMS Fault ID28 ==
  State : Inport
  Bus Creator1 : BusCreator  Inputs=2  OutDataTypeStr=Bus: BD_TCMSSystem_Out_Vehicle_Display_Message  NonVirtualBus=on
  Constant : Constant  Value=MessageID
  Data Type Conversion : DataTypeConversion
  Message : Outport  VectorParamsAs1DForOutWhenUnconnected=off
  wires:
  Bus Creator1/1 -> Message/1
  State/1 -> Data Type Conversion/1
  Constant/1 -> Bus Creator1/1  "MessageID"
  Data Type Conversion/1 -> Bus Creator1/2  "MessageStatus"

== system TCMSSystem/TCMSSystemPerVehicle/EnabledTCMSVehicle/OutputsPacking/TCMSDisplayOutputs/TCMSMessageEvents/ElectricalSystemFaults/Associated TCMS Fault ID29 ==
  State : Inport
  Bus Creator1 : BusCreator  Inputs=2  OutDataTypeStr=Bus: BD_TCMSSystem_Out_Vehicle_Display_Message  NonVirtualBus=on
  Constant : Constant  Value=MessageID
  Data Type Conversion : DataTypeConversion
  Message : Outport  VectorParamsAs1DForOutWhenUnconnected=off
  wires:
  Data Type Conversion/1 -> Bus Creator1/2  "MessageStatus"
  Constant/1 -> Bus Creator1/1  "MessageID"
  State/1 -> Data Type Conversion/1
  Bus Creator1/1 -> Message/1

== system TCMSSystem/TCMSSystemPerVehicle/EnabledTCMSVehicle/OutputsPacking/TCMSDisplayOutputs/TCMSMessageEvents/ElectricalSystemFaults/Associated TCMS Fault ID3 ==
  State : Inport
  Bus Creator1 : BusCreator  Inputs=2  OutDataTypeStr=Bus: BD_TCMSSystem_Out_Vehicle_Display_Message  NonVirtualBus=on
  Constant : Constant  Value=MessageID
  Data Type Conversion : DataTypeConversion
  Message : Outport  VectorParamsAs1DForOutWhenUnconnected=off
  wires:
  Bus Creator1/1 -> Message/1
  State/1 -> Data Type Conversion/1
  Constant/1 -> Bus Creator1/1  "MessageID"
  Data Type Conversion/1 -> Bus Creator1/2  "MessageStatus"

== system TCMSSystem/TCMSSystemPerVehicle/EnabledTCMSVehicle/OutputsPacking/TCMSDisplayOutputs/TCMSMessageEvents/ElectricalSystemFaults/Associated TCMS Fault ID30 ==
  State : Inport
  Bus Creator1 : BusCreator  Inputs=2  OutDataTypeStr=Bus: BD_TCMSSystem_Out_Vehicle_Display_Message  NonVirtualBus=on
  Constant : Constant  Value=MessageID
  Data Type Conversion : DataTypeConversion
  Message : Outport  VectorParamsAs1DForOutWhenUnconnected=off
  wires:
  Bus Creator1/1 -> Message/1
  State/1 -> Data Type Conversion/1
  Constant/1 -> Bus Creator1/1  "MessageID"
  Data Type Conversion/1 -> Bus Creator1/2  "MessageStatus"

== system TCMSSystem/TCMSSystemPerVehicle/EnabledTCMSVehicle/OutputsPacking/TCMSDisplayOutputs/TCMSMessageEvents/ElectricalSystemFaults/Associated TCMS Fault ID31 ==
  State : Inport
  Bus Creator1 : BusCreator  Inputs=2  OutDataTypeStr=Bus: BD_TCMSSystem_Out_Vehicle_Display_Message  NonVirtualBus=on
  Constant : Constant  Value=MessageID
  Data Type Conversion : DataTypeConversion
  Message : Outport  VectorParamsAs1DForOutWhenUnconnected=off
  wires:
  Data Type Conversion/1 -> Bus Creator1/2  "MessageStatus"
  Constant/1 -> Bus Creator1/1  "MessageID"
  State/1 -> Data Type Conversion/1
  Bus Creator1/1 -> Message/1

== system TCMSSystem/TCMSSystemPerVehicle/EnabledTCMSVehicle/OutputsPacking/TCMSDisplayOutputs/TCMSMessageEvents/ElectricalSystemFaults/Associated TCMS Fault ID32 ==
  State : Inport
  Bus Creator1 : BusCreator  Inputs=2  OutDataTypeStr=Bus: BD_TCMSSystem_Out_Vehicle_Display_Message  NonVirtualBus=on
  Constant : Constant  Value=MessageID
  Data Type Conversion : DataTypeConversion
  Message : Outport  VectorParamsAs1DForOutWhenUnconnected=off
  wires:
  Data Type Conversion/1 -> Bus Creator1/2  "MessageStatus"
  Constant/1 -> Bus Creator1/1  "MessageID"
  State/1 -> Data Type Conversion/1
  Bus Creator1/1 -> Message/1

== system TCMSSystem/TCMSSystemPerVehicle/EnabledTCMSVehicle/OutputsPacking/TCMSDisplayOutputs/TCMSMessageEvents/ElectricalSystemFaults/Associated TCMS Fault ID33 ==
  State : Inport
  Bus Creator1 : BusCreator  Inputs=2  OutDataTypeStr=Bus: BD_TCMSSystem_Out_Vehicle_Display_Message  NonVirtualBus=on
  Constant : Constant  Value=MessageID
  Data Type Conversion : DataTypeConversion
  Message : Outport  VectorParamsAs1DForOutWhenUnconnected=off
  wires:
  Bus Creator1/1 -> Message/1
  State/1 -> Data Type Conversion/1
  Constant/1 -> Bus Creator1/1  "MessageID"
  Data Type Conversion/1 -> Bus Creator1/2  "MessageStatus"

== system TCMSSystem/TCMSSystemPerVehicle/EnabledTCMSVehicle/OutputsPacking/TCMSDisplayOutputs/TCMSMessageEvents/ElectricalSystemFaults/Associated TCMS Fault ID34 ==
  State : Inport
  Bus Creator1 : BusCreator  Inputs=2  OutDataTypeStr=Bus: BD_TCMSSystem_Out_Vehicle_Display_Message  NonVirtualBus=on
  Constant : Constant  Value=MessageID
  Data Type Conversion : DataTypeConversion
  Message : Outport  VectorParamsAs1DForOutWhenUnconnected=off
  wires:
  Bus Creator1/1 -> Message/1
  State/1 -> Data Type Conversion/1
  Constant/1 -> Bus Creator1/1  "MessageID"
  Data Type Conversion/1 -> Bus Creator1/2  "MessageStatus"

== system TCMSSystem/TCMSSystemPerVehicle/EnabledTCMSVehicle/OutputsPacking/TCMSDisplayOutputs/TCMSMessageEvents/ElectricalSystemFaults/Associated TCMS Fault ID35 ==
  State : Inport
  Bus Creator1 : BusCreator  Inputs=2  OutDataTypeStr=Bus: BD_TCMSSystem_Out_Vehicle_Display_Message  NonVirtualBus=on
  Constant : Constant  Value=MessageID
  Data Type Conversion : DataTypeConversion
  Message : Outport  VectorParamsAs1DForOutWhenUnconnected=off
  wires:
  Data Type Conversion/1 -> Bus Creator1/2  "MessageStatus"
  Constant/1 -> Bus Creator1/1  "MessageID"
  State/1 -> Data Type Conversion/1
  Bus Creator1/1 -> Message/1

== system TCMSSystem/TCMSSystemPerVehicle/EnabledTCMSVehicle/OutputsPacking/TCMSDisplayOutputs/TCMSMessageEvents/ElectricalSystemFaults/Associated TCMS Fault ID36 ==
  State : Inport
  Bus Creator1 : BusCreator  Inputs=2  OutDataTypeStr=Bus: BD_TCMSSystem_Out_Vehicle_Display_Message  NonVirtualBus=on
  Constant : Constant  Value=MessageID
  Data Type Conversion : DataTypeConversion
  Message : Outport  VectorParamsAs1DForOutWhenUnconnected=off
  wires:
  Bus Creator1/1 -> Message/1
  State/1 -> Data Type Conversion/1
  Constant/1 -> Bus Creator1/1  "MessageID"
  Data Type Conversion/1 -> Bus Creator1/2  "MessageStatus"
